simulink model "untitled"  (R2018b)
settings: Solver=FixedStepAuto  StartTime=0.0  StopTime=10  FixedStep=1  RelTol=1e-3
settings Model: Creator=jianhuili  LastModifiedBy=jianhuili

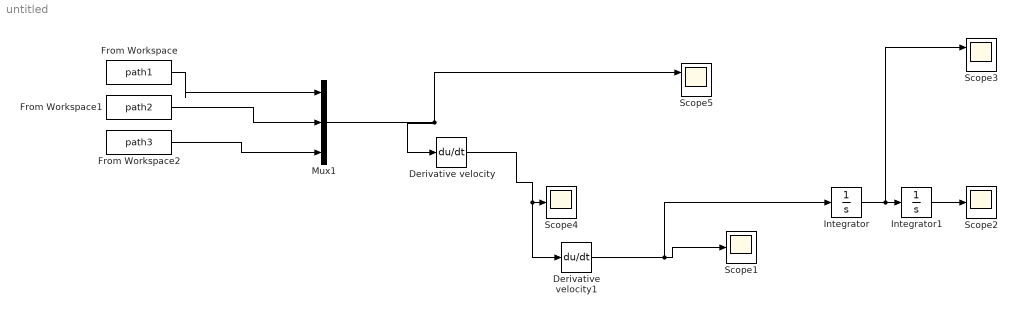
== system untitled ==
  Derivative velocity : Derivative
  Derivative velocity1 : Derivative
  From Workspace : FromWorkspace  VariableName=path1  SampleTime=0.001  Interpolate=off  OutputAfterFinalValue=Holding final value
  From Workspace1 : FromWorkspace  VariableName=path2  SampleTime=0.001  Interpolate=off  OutputAfterFinalValue=Holding final value
  From Workspace2 : FromWorkspace  VariableName=path3  SampleTime=0.001  Interpolate=off  OutputAfterFinalValue=Holding final value
  Integrator : Integrator
  Integrator1 : Integrator
  Mux1 : Mux  Inputs=3
  Scope1 : Scope
  Scope2 : Scope
  Scope3 : Scope  NumInputPorts=2
  Scope4 : Scope
  Scope5 : Scope  NumInputPorts=2
  wires:
  Mux1/1 -> Derivative velocity/1, Scope5/1
  Derivative velocity/1 -> Scope4/1, Derivative velocity1/1
  Derivative velocity1/1 -> Integrator/1, Scope1/1
  Integrator/1 -> Scope3/1, Integrator1/1
  From Workspace2/1 -> Mux1/3
  From Workspace/1 -> Mux1/1
  From Workspace1/1 -> Mux1/2
  Integrator1/1 -> Scope2/1
